simulink model "sine_squ_plus_cosine_sqr_1"  (R2024b)
settings: Solver=VariableStepAuto  StartTime=0.0  StopTime=10.0  MaxStep=0.0001  RelTol=1e-3
settings Model: Creator=admin  LastModifiedBy=admin

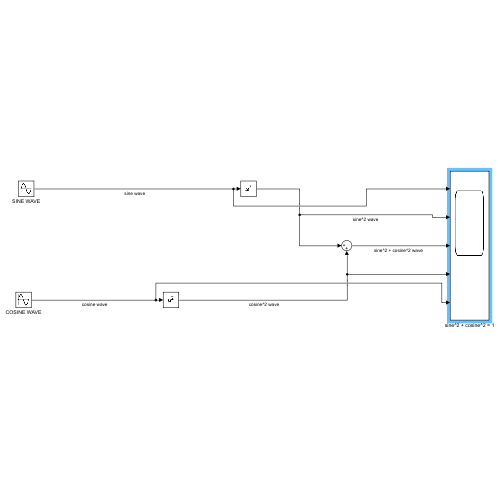
[thumbnail: Simulink's stored preview of the top-level diagram]
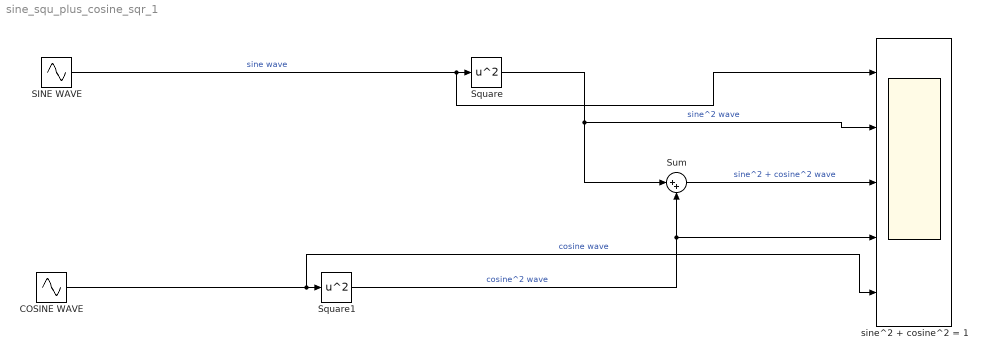
== system sine_squ_plus_cosine_sqr_1 ==
  COSINE WAVE : Sin  Phase=pi/2  SampleTime=0
  SINE WAVE : Sin  SampleTime=0
  Square : Math  Operator=square
  Square1 : Math  Operator=square
  Sum : Sum  Inputs=|++
  sine^2 + cosine^2 = 1 : Scope  NumInputPorts=5
  wires:
  SINE WAVE/1 -> sine^2 + cosine^2 = 1/1, Square/1  "sine wave"
  COSINE WAVE/1 -> sine^2 + cosine^2 = 1/5, Square1/1  "cosine wave"
  Square1/1 -> sine^2 + cosine^2 = 1/4, Sum/2  "cosine^2 wave"
  Square/1 -> sine^2 + cosine^2 = 1/2, Sum/1  "sine^2 wave"
  Sum/1 -> sine^2 + cosine^2 = 1/3  "sine^2 + cosine^2 wave"
